simulink model "ControlloreNonLineare"  (R2024b)
settings: Solver=ode1be  StartTime=0.0  StopTime=10  RelTol=1e-3
settings Model: PacingRate=0.100000  Creator=feder  LastModifiedBy=Salvatore

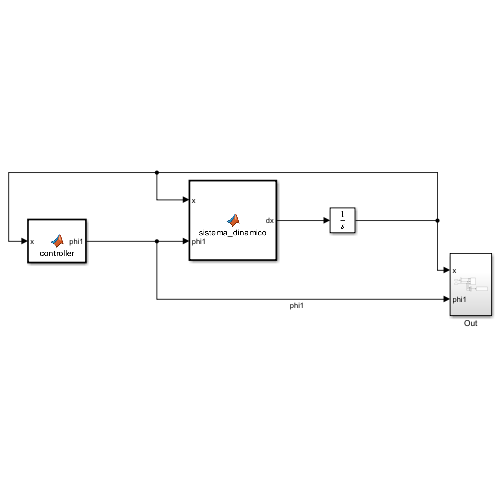
[thumbnail: Simulink's stored preview of the top-level diagram]
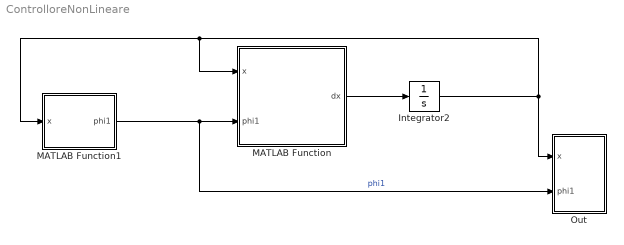
== system ControlloreNonLineare ==
  Integrator2 : Integrator  InitialCondition=[2;2]
  MATLAB Function : MATLAB Function  TreatAsAtomicUnit=on
  MATLAB Function1 : MATLAB Function  TreatAsAtomicUnit=on
  Out : Subsystem
  wires:
  MATLAB Function/1(dx) -> Integrator2/1
  Integrator2/1 -> Out/1(x), MATLAB Function1/1("x "), MATLAB Function/1(x)
  MATLAB Function1/1(phi1) -> Out/2(phi1), MATLAB Function/2(phi1)  "phi1"

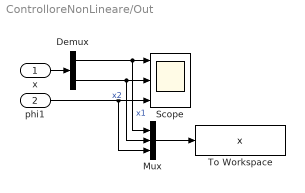
== system ControlloreNonLineare/Out ==
  x : Inport
  phi1 : Inport  Port=2
  Demux : Demux  Outputs=2
  Mux : Mux  Inputs=3
  Scope : Scope  NumInputPorts=3
  To Workspace : ToWorkspace  VariableName=x  SampleTime=-1
      settings: Save2DSignal=2-D array (concatenate along first dimension)
  wires:
  x/1 -> Demux/1
  Demux/1 -> Mux/1, Scope/1  "x1"
  phi1/1 -> Mux/3, Scope/3
  Demux/2 -> Mux/2, Scope/2  "x2"
  Mux/1 -> To Workspace/1

== matlab function ControlloreNonLineare/MATLAB Function1 ==
  data: phi1 output; x input
function phi1 = controller(x) % Parametri
    %Guadagno del controllore
    k1=2;

    %unpack
    x1 = x(1);
    x2 = x(2);
    
    %Controllore
    phi1=-x2^3-2*x1^2*x2-k1*x2;
end

== matlab function ControlloreNonLineare/MATLAB Function ==
  data: dx output; x input; phi1 input
function dx = sistema_dinamico(x, phi1)
    % Ingressi del sistema
    x_1 = x(1);
    x_2 = x(2);
    x_3 = phi1;

    % Derivate
    dx1 = x_1 * (x_1^2 + x_2^2 - 4) - x_2-x_1^3;
    dx2 = x_2 * (x_1^2 + x_2^2 - 4) + x_1 + x_3;
    
    dx = [dx1; dx2];
end
